simulink model "RNC_S"  (R2019b)
settings: Solver=VariableStepAuto  StartTime=0.0  StopTime=10.0  RelTol=1e-3
values from neighbouring files (symbols this model uses):
  K = [-5 -2;-1 -6]    [out.m]
  k = [-4 -2;-1 -5]    [out.m]
  proportion = stepsize/sampleperiod*100-0.001    (= 99.999)    [out.m]
  sampleperiod = 0.04    [out.m]
  stepsize = 0.04    [out.m]
settings Model: Creator=techman  LastModifiedBy=techman
settings DataIOCC: ReturnWorkspaceOutputs=off

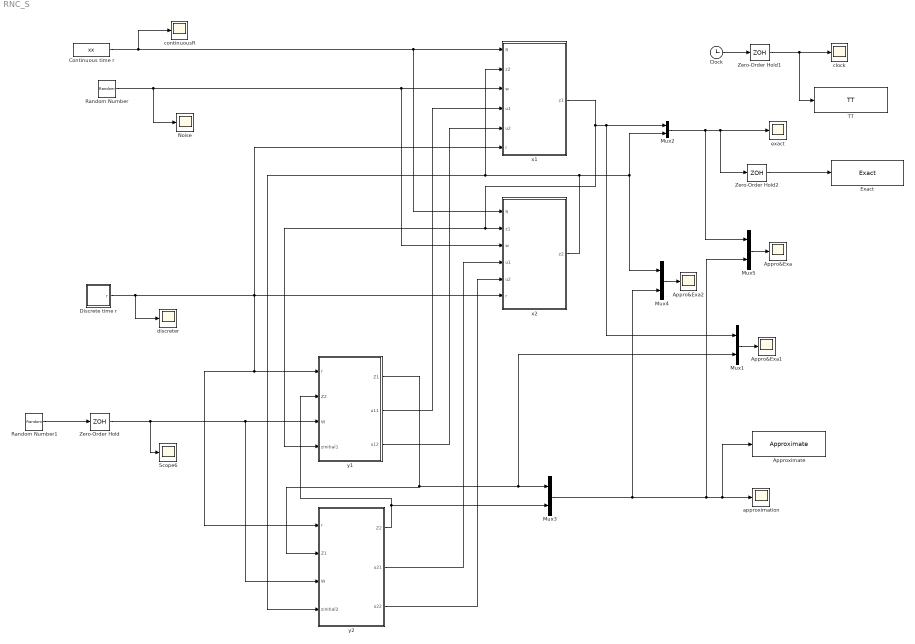
== system RNC_S ==
  " Exact" : ToWorkspace  VariableName=Exact  SampleTime=-1
  " TT" : ToWorkspace  VariableName=TT  SampleTime=-1
  Appro&Exa : Scope
  Appro&Exa1 : Scope
  Appro&Exa2 : Scope
  Approximate : ToWorkspace  VariableName=Approximate  SampleTime=-1
  Clock : Clock
  Continuous time r : FromWorkspace  VariableName=xx  SampleTime=0
  Discrete time r : Subsystem
  Mux{1..5} (5 alike) : Mux  Inputs=2
  Noise : Scope
  Random Number : RandomNumber  Variance=0.1  SampleTime=0.001
  Random Number1 : RandomNumber  Variance=0.1  SampleTime=0.001
  Scope6 : Scope
  Zero-Order Hold : ZeroOrderHold  SampleTime=stepsize
  Zero-Order Hold1 : ZeroOrderHold  SampleTime=0.001
  Zero-Order Hold2 : ZeroOrderHold  SampleTime=0.001
  approximation : Scope
  clock : Scope
  continuousR : Scope
  discreter : Scope
  exact : Scope
  x1 : Subsystem
  x2 : Subsystem
  y1 : Subsystem
  y2 : Subsystem
  wires:
  y2/2(u21) -> x2/4(u1)
  y1/1(Z1) -> Mux1/2, Mux3/1, y2/2(Z1)
  Zero-Order Hold/1 -> Scope6/1, y2/3(W), y1/3(W)
  Mux1/1 -> Appro&Exa1/1
  x2/1(z2) -> Mux2/2, Mux4/1, x1/2(z2), y2/4(zinitial2)
  Discrete time r/1(r) -> discreter/1, y2/1(r), y1/1(r), x2/6(r), x1/6(r)
  Mux2/1 -> Zero-Order Hold2/1, exact/1, Mux5/1
  Zero-Order Hold1/1 -> " TT"/1, clock/1
  y1/2(u11) -> x1/4(u1)
  y1/3(u12) -> x1/5(u2)
  Mux5/1 -> Appro&Exa/1
  x1/1(z1) -> Mux1/1, Mux2/1, y1/4(zinitial1), x2/2(z1)
  y2/1(Z2) -> y1/2(Z2), Mux3/2
  Mux3/1 -> Mux4/2, Mux5/2, Approximate/1, approximation/1
  Random Number/1 -> Noise/1, x1/3(w), x2/3(w)
  Clock/1 -> Zero-Order Hold1/1
  Mux4/1 -> Appro&Exa2/1
  y2/3(u22) -> x2/5(u2)
  Random Number1/1 -> Zero-Order Hold/1
  Continuous time r/1 -> x1/1(R), x2/1(R), continuousR/1
  Zero-Order Hold2/1 -> " Exact"/1

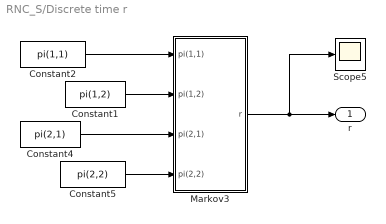
== system RNC_S/Discrete time r ==
  Constant1 : Constant  Value=pi(1,2)
  Constant2 : Constant  Value=pi(1,1)
  Constant4 : Constant  Value=pi(2,1)
  Constant5 : Constant  Value=pi(2,2)
  Markov3 : Subsystem
  Scope5 : Scope
  r : Outport  VectorParamsAs1DForOutWhenUnconnected=off
  wires:
  Constant1/1 -> Markov3/2(pi(1,2))
  Constant2/1 -> Markov3/1(pi(1,1))
  Constant4/1 -> Markov3/3(pi(2,1))
  Constant5/1 -> Markov3/4(pi(2,2))
  Markov3/1(r) -> r/1, Scope5/1

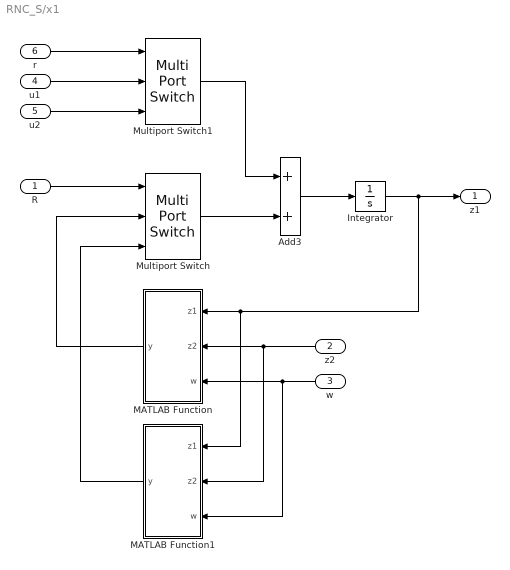
== system RNC_S/x1 ==
  R : Inport
  z2 : Inport  Port=2
  w : Inport  Port=3
  u1 : Inport  Port=4
  u2 : Inport  Port=5
  r : Inport  Port=6
  Add3 : Sum
  Integrator : Integrator  InitialCondition=-3
  MATLAB Function : MATLAB Function  TreatAsAtomicUnit=on
  MATLAB Function1 : MATLAB Function  TreatAsAtomicUnit=on
  Multiport Switch : MultiPortSwitch  Inputs=2
  Multiport Switch1 : MultiPortSwitch  Inputs=2
  z1 : Outport  VectorParamsAs1DForOutWhenUnconnected=off
  wires:
  R/1 -> Multiport Switch/1
  Integrator/1 -> MATLAB Function1/1(z1), MATLAB Function/1(z1), z1/1
  r/1 -> Multiport Switch1/1
  u2/1 -> Multiport Switch1/3
  u1/1 -> Multiport Switch1/2
  Multiport Switch1/1 -> Add3/1
  Multiport Switch/1 -> Add3/2
  Add3/1 -> Integrator/1
  w/1 -> MATLAB Function1/3(w), MATLAB Function/3(w)
  z2/1 -> MATLAB Function1/2(z2), MATLAB Function/2(z2)
  MATLAB Function/1(y) -> Multiport Switch/2
  MATLAB Function1/1(y) -> Multiport Switch/3

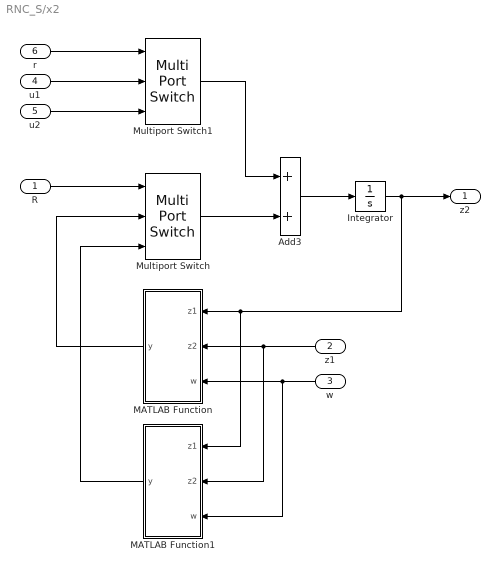
== system RNC_S/x2 ==
  R : Inport
  z1 : Inport  Port=2
  w : Inport  Port=3
  u1 : Inport  Port=4
  u2 : Inport  Port=5
  r : Inport  Port=6
  Add3 : Sum
  Integrator : Integrator  InitialCondition=3
  MATLAB Function : MATLAB Function  TreatAsAtomicUnit=on
  MATLAB Function1 : MATLAB Function  TreatAsAtomicUnit=on
  Multiport Switch : MultiPortSwitch  Inputs=2
  Multiport Switch1 : MultiPortSwitch  Inputs=2
  z2 : Outport  VectorParamsAs1DForOutWhenUnconnected=off
  wires:
  Add3/1 -> Integrator/1
  r/1 -> Multiport Switch1/1
  MATLAB Function1/1(y) -> Multiport Switch/3
  z1/1 -> MATLAB Function1/2(z2), MATLAB Function/2(z2)
  Multiport Switch1/1 -> Add3/1
  MATLAB Function/1(y) -> Multiport Switch/2
  w/1 -> MATLAB Function1/3(w), MATLAB Function/3(w)
  R/1 -> Multiport Switch/1
  u1/1 -> Multiport Switch1/2
  Integrator/1 -> MATLAB Function1/1(z1), MATLAB Function/1(z1), z2/1
  u2/1 -> Multiport Switch1/3
  Multiport Switch/1 -> Add3/2

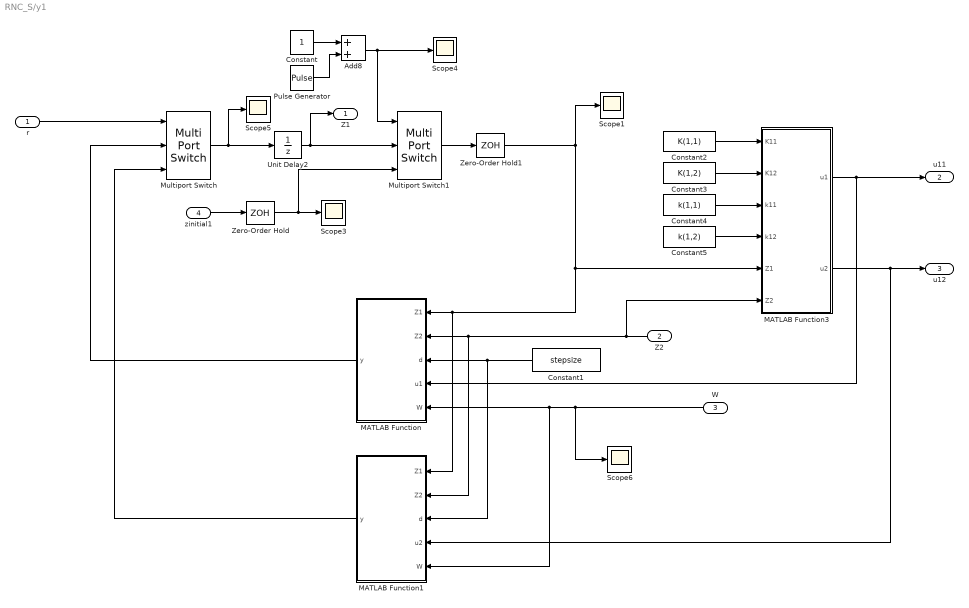
== system RNC_S/y1 ==
  r : Inport
  Z2 : Inport  Port=2
  W : Inport  Port=3
  zinitial1 : Inport  Port=4
  Add8 : Sum
  Constant : Constant
  Constant1 : Constant  Value=stepsize
  Constant2 : Constant  Value=K(1,1)
  Constant3 : Constant  Value=K(1,2)
  Constant4 : Constant  Value=k(1,1)
  Constant5 : Constant  Value=k(1,2)
  MATLAB Function : MATLAB Function  TreatAsAtomicUnit=on
  MATLAB Function1 : MATLAB Function  TreatAsAtomicUnit=on
  MATLAB Function3 : MATLAB Function  TreatAsAtomicUnit=on
  Multiport Switch : MultiPortSwitch  Inputs=2
  Multiport Switch1 : MultiPortSwitch  Inputs=2
  Pulse Generator : DiscretePulseGenerator  PulseType=Time based  Period=sampleperiod  PulseWidth=proportion
  Scope{1,3..6} (5 alike) : Scope
  Unit Delay2 : UnitDelay  InitialCondition=-3  InputProcessing=Columns as channels (frame based)  SampleTime=stepsize  HasFrameUpgradeWarning=on
  Zero-Order Hold : ZeroOrderHold  SampleTime=sampleperiod
  Zero-Order Hold1 : ZeroOrderHold  SampleTime=stepsize
  Z1 : Outport  VectorParamsAs1DForOutWhenUnconnected=off
  u11 : Outport  Port=2  VectorParamsAs1DForOutWhenUnconnected=off
  u12 : Outport  Port=3  VectorParamsAs1DForOutWhenUnconnected=off
  wires:
  r/1 -> Multiport Switch/1
  zinitial1/1 -> Zero-Order Hold/1
  Pulse Generator/1 -> Add8/2
  Constant/1 -> Add8/1
  Add8/1 -> Multiport Switch1/1, Scope4/1
  Zero-Order Hold/1 -> Multiport Switch1/3, Scope3/1
  Multiport Switch/1 -> Unit Delay2/1, Scope5/1
  W/1 -> MATLAB Function1/5(W), MATLAB Function/5(W), Scope6/1
  Constant1/1 -> MATLAB Function/3(d), MATLAB Function1/3(d)
  MATLAB Function/1(y) -> Multiport Switch/2
  MATLAB Function1/1(y) -> Multiport Switch/3
  Z2/1 -> MATLAB Function3/6(Z2), MATLAB Function/2(Z2), MATLAB Function1/2(Z2)
  Constant2/1 -> MATLAB Function3/1(K11)
  Constant3/1 -> MATLAB Function3/2(K12)
  Constant4/1 -> MATLAB Function3/3(k11)
  Constant5/1 -> MATLAB Function3/4(k12)
  MATLAB Function3/1(u1) -> MATLAB Function/4(u1), u11/1
  MATLAB Function3/2(u2) -> MATLAB Function1/4(u2), u12/1
  Multiport Switch1/1 -> Zero-Order Hold1/1
  Unit Delay2/1 -> Multiport Switch1/2, Z1/1
  Zero-Order Hold1/1 -> MATLAB Function3/5(Z1), MATLAB Function1/1(Z1), MATLAB Function/1(Z1), Scope1/1

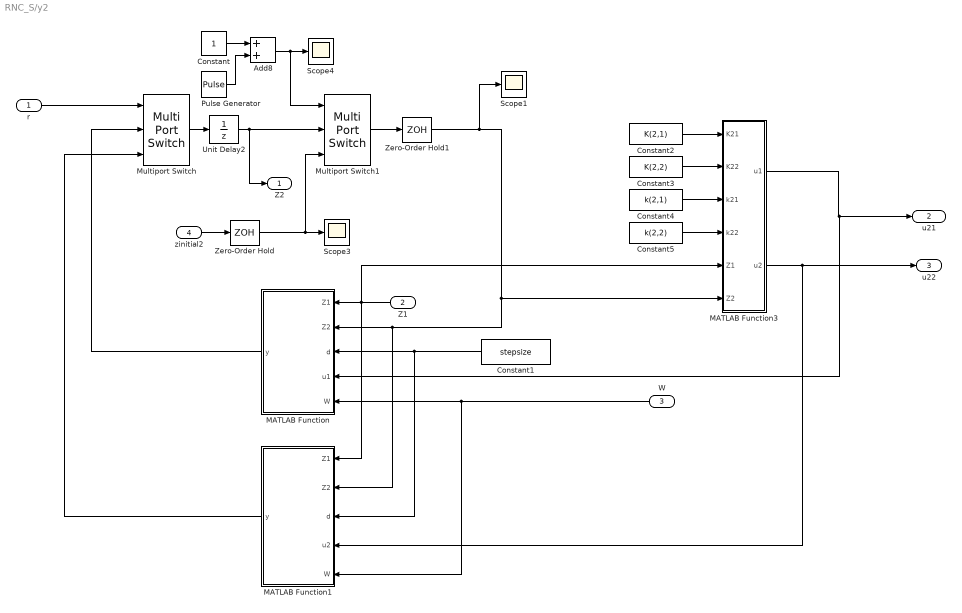
== system RNC_S/y2 ==
  r : Inport
  Z1 : Inport  Port=2
  W : Inport  Port=3
  zinitial2 : Inport  Port=4
  Add8 : Sum
  Constant : Constant
  Constant1 : Constant  Value=stepsize
  Constant2 : Constant  Value=K(2,1)
  Constant3 : Constant  Value=K(2,2)
  Constant4 : Constant  Value=k(2,1)
  Constant5 : Constant  Value=k(2,2)
  MATLAB Function : MATLAB Function  TreatAsAtomicUnit=on
  MATLAB Function1 : MATLAB Function  TreatAsAtomicUnit=on
  MATLAB Function3 : MATLAB Function  TreatAsAtomicUnit=on
  Multiport Switch : MultiPortSwitch  Inputs=2
  Multiport Switch1 : MultiPortSwitch  Inputs=2
  Pulse Generator : DiscretePulseGenerator  PulseType=Time based  Period=sampleperiod  PulseWidth=proportion
  Scope1 : Scope
  Scope3 : Scope
  Scope4 : Scope
  Unit Delay2 : UnitDelay  InitialCondition=3  InputProcessing=Columns as channels (frame based)  SampleTime=stepsize  HasFrameUpgradeWarning=on
  Zero-Order Hold : ZeroOrderHold  SampleTime=sampleperiod
  Zero-Order Hold1 : ZeroOrderHold  SampleTime=stepsize
  Z2 : Outport  VectorParamsAs1DForOutWhenUnconnected=off
  u21 : Outport  Port=2  VectorParamsAs1DForOutWhenUnconnected=off
  u22 : Outport  Port=3  VectorParamsAs1DForOutWhenUnconnected=off
  wires:
  r/1 -> Multiport Switch/1
  Pulse Generator/1 -> Add8/2
  Add8/1 -> Multiport Switch1/1, Scope4/1
  Constant/1 -> Add8/1
  zinitial2/1 -> Zero-Order Hold/1
  Zero-Order Hold/1 -> Multiport Switch1/3, Scope3/1
  Constant1/1 -> MATLAB Function1/3(d), MATLAB Function/3(d)
  W/1 -> MATLAB Function1/5(W), MATLAB Function/5(W)
  MATLAB Function/1(y) -> Multiport Switch/2
  MATLAB Function1/1(y) -> Multiport Switch/3
  Z1/1 -> MATLAB Function3/5(Z1), MATLAB Function1/1(Z1), MATLAB Function/1(Z1)
  Constant5/1 -> MATLAB Function3/4(k22)
  Constant3/1 -> MATLAB Function3/2(K22)
  Constant4/1 -> MATLAB Function3/3(k21)
  Constant2/1 -> MATLAB Function3/1(K21)
  MATLAB Function3/1(u1) -> MATLAB Function/4(u1), u21/1
  MATLAB Function3/2(u2) -> MATLAB Function1/4(u2), u22/1
  Multiport Switch1/1 -> Zero-Order Hold1/1
  Multiport Switch/1 -> Unit Delay2/1
  Unit Delay2/1 -> Z2/1, Multiport Switch1/2
  Zero-Order Hold1/1 -> Scope1/1, MATLAB Function3/6(Z2), MATLAB Function1/2(Z2), MATLAB Function/2(Z2)

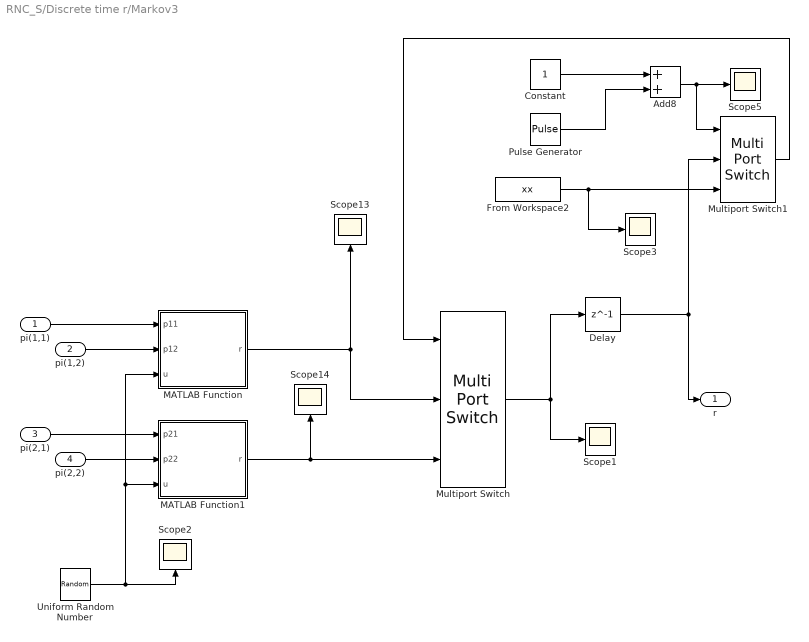
== system RNC_S/Discrete time r/Markov3 ==
  pi(1,1) : Inport
  pi(1,2) : Inport  Port=2
  pi(2,1) : Inport  Port=3
  pi(2,2) : Inport  Port=4
  Add8 : Sum
  Constant : Constant
  Delay : Delay  DelayLength=1  InitialCondition=1  SampleTime=sampleperiod
  From Workspace2 : FromWorkspace  VariableName=xx  SampleTime=0
  MATLAB Function : MATLAB Function  TreatAsAtomicUnit=on
  MATLAB Function1 : MATLAB Function  TreatAsAtomicUnit=on
  Multiport Switch : MultiPortSwitch  Inputs=2
  Multiport Switch1 : MultiPortSwitch  Inputs=2
  Pulse Generator : DiscretePulseGenerator  PulseType=Time based  Period=sampleperiod  PulseWidth=10
  Scope{1..3,5,13..14} (6 alike) : Scope
  Uniform Random Number : UniformRandomNumber  Minimum=0  SampleTime=0.01
  r : Outport  VectorParamsAs1DForOutWhenUnconnected=off
  wires:
  pi(2,2)/1 -> MATLAB Function1/2(p22)
  pi(1,1)/1 -> MATLAB Function/1(p11)
  pi(1,2)/1 -> MATLAB Function/2(p12)
  MATLAB Function/1(r) -> Scope13/1, Multiport Switch/2
  pi(2,1)/1 -> MATLAB Function1/1(p21)
  Multiport Switch/1 -> Delay/1, Scope1/1
  Uniform Random Number/1 -> Scope2/1, MATLAB Function/3(u), MATLAB Function1/3(u)
  MATLAB Function1/1(r) -> Multiport Switch/3, Scope14/1
  From Workspace2/1 -> Scope3/1, Multiport Switch1/3
  Pulse Generator/1 -> Add8/2
  Constant/1 -> Add8/1
  Add8/1 -> Multiport Switch1/1, Scope5/1
  Delay/1 -> Multiport Switch1/2, r/1
  Multiport Switch1/1 -> Multiport Switch/1

== matlab function RNC_S/x1/MATLAB Function ==
  data: z1 input; z2 input; w input; y output
function y = fcn(z1,z2,w)
%#codegen
    y = 5.*z1.*sin(z2)+3.*z2+sin(z1).*w;
end

== matlab function RNC_S/Discrete time r/Markov3/MATLAB Function ==
  data: p11 input; p12 input; u input; r output
function r = fcn(p11,p12,u)
%#codegen
if u<p11
    r = 1;
else
    r = 2;
end

== matlab function RNC_S/Discrete time r/Markov3/MATLAB Function1 ==
  data: p21 input; p22 input; u input; r output
function r = fcn(p21,p22,u)
%#codegen
if u<p21
    r = 1;
else
    r = 2;
end

== matlab function RNC_S/x1/MATLAB Function1 ==
  data: z1 input; z2 input; w input; y output
function y = fcn(z1,z2,w)
%#codegen
    y = 2.*z1.*cos(z2)+4.*z2+z1.*w;
end

== matlab function RNC_S/x2/MATLAB Function ==
  data: z1 input; z2 input; w input; y output
function y = fcn(z1,z2,w)
%#codegen
    y = 4.*sin(z1).*sqrt((1+z2).*(1+z2))+z2.*w;
end

== matlab function RNC_S/x2/MATLAB Function1 ==
  data: z1 input; z2 input; w input; y output
function y = fcn(z1,z2,w)
%#codegen
    y = 5.*z2./(1+z1.*z1)+sin(z2).*w;
end

== matlab function RNC_S/y1/MATLAB Function ==
  data: Z1 input; Z2 input; d input; u1 input; W input; y output
function y = fcn(Z1,Z2,d,u1,W)
%#codegen
    y = Z1+d.*(5.*Z1*sin(Z2)+3.*Z2+u1)+sin(Z1).*W;
end

== matlab function RNC_S/y1/MATLAB Function1 ==
  data: Z1 input; Z2 input; d input; y output; u2 input; W input
function y = fcn(Z1,Z2,d,u2,W)
%#codegen
    y = Z1+d.*(2.*Z1.*cos(Z2)+4.*Z2+u2)+Z1.*W;
end

== matlab function RNC_S/y2/MATLAB Function ==
  data: Z1 input; Z2 input; d input; y output; u1 input; W input
function y = fcn(Z1,Z2,d,u1,W)
%#codegen
    y = Z2+d.*(4.*sin(Z1).*sqrt((1+Z2).*(1+Z2))+u1)+Z2.*W;
end

== matlab function RNC_S/y2/MATLAB Function1 ==
  data: Z1 input; Z2 input; d input; y output; u2 input; W input
function y = fcn(Z1,Z2,d,u2,W)
%#codegen
    y = Z2+d.*(5.*Z2/(1+Z1.*Z1)+u2)+sin(Z2).*W;
end

== matlab function RNC_S/y2/MATLAB Function3 ==
  data: K21 input; K22 input; k21 input; k22 input; Z1 input; Z2 input; u1 output; u2 output
function [u1,u2] = fcn(K21,K22,k21,k22,Z1,Z2)
%#codegen
    u1 = K21.*Z1 + K22.*Z2;
    u2 = k21.*Z1 + k22.*Z2;
end

== matlab function RNC_S/y1/MATLAB Function3 ==
  data: K11 input; K12 input; k11 input; k12 input; Z1 input; Z2 input; u1 output; u2 output
function [u1,u2] = fcn(K11,K12,k11,k12,Z1,Z2)
%#codegen
    u1 = K11.*Z1 + K12.*Z2;
    u2 = k11.*Z1 + k12.*Z2;
end
